simulink model "Main_ekart"  (R2021b)
settings: Solver=FixedStepAuto  StartTime=0.0  StopTime=inf  FixedStep=1/500  RelTol=1e-3  EnableMultiTasking=on
values from neighbouring files (symbols this model uses):
  a = [1 -2.62355180661 2.31468258109 -0.685535977285]    [IMU_filt_100Hz.mat]    (also in IMU_filt_500Hz.mat = [1 -2.92460623545 2.85202781859 -0.92736996835])
  angles = [0 4.9 5 10 15 20 25 30 35 40]    [CreateAllControllers.m]
  b = [0.000699349649901 0.0020980489497 0.0020980489497 0.000699349649901]    [IMU_filt_100Hz.mat]    (also in IMU_filt_500Hz.mat = [6.45184912909e-06 1.93555473873e-05 1.93555473873e-05 6.451)
  D = (DMFx+DMFy)/2    (= 1.2194)    [kart_parameters2.m]
  gear_ratio = 3.2    [kart_parameters2.m]
  L = sys*C    [build_controller_PI.m]    (also in kart_parameters2.m = 1.042)
  newcurrent = [-186.423 -186.283922965 -186.14484593 -186.005768895 -185.866691861 -185.727614826 -185.588537791 -185.449460756 -185.310383721 -185.171306686 -185.032229652 -184.893152617 ... (1000 elements, 1x1000)]    [Torque_map.mat]
  newtorque = [-28.1755 -28.1190925926 -28.0626851852 -28.0062777778 -27.9498703704 -27.893462963 -27.8370555556 -27.7806481481 -27.7242407407 -27.6678333333 -27.6114259259 -27.5550185185 ... (1000 elements, 1x1000)]    [Torque_map.mat]
  percent = [0 0.1001001001 0.2002002002 0.3003003003 0.4004004004 0.500500500501 0.600600600601 0.700700700701 0.800800800801 0.900900900901 1.001001001 1.1011011011 ... (1000 elements, 1x1000)]    [Torque_accel.mat]
  speeds = [0 19.9 20 30 40]    [CreateAllControllers.m]
  table_i = [zeros(1,10) ... (first row only)    [CreateAllControllers.m]
  table_p = [zeros(1, 10) ... (first row only)    [CreateAllControllers.m]
  torque = [0.1025 0.130601101101 0.158702202202 0.186803303303 0.214904404404 0.243005505506 0.271106606607 0.299207707708 0.327308808809 0.35540990991 0.383511011011 0.411612112112 ... (1000 elements, 1x1000)]    [Torque_accel.mat]
libraries: simulink x50, mcp2515lib x46, etargetslib x4, svdutilitieslib x3, cstblocks x2, slpidlib x1
(part 2 of 4)

== system Main_ekart/Receive_CAN/Subsystem6 ==
  CAN_Received : Inport
  CAN_EXT : Inport  Port=2
  CAN_ID : Inport  Port=3
  CAN_DLC : Inport  Port=4
  CAN_DATA : Inport  Port=5
  AND : Logic  Inputs=4  IconShape=distinctive  AllPortsSameDT=off  OutDataTypeStr=boolean
  Compare To Desired DLC : simulink/Logic and Bit Operations/Compare To Constant  relop===  const=DLC  OutDataTypeStr=boolean
  Compare To Desired DLC1 : simulink/Logic and Bit Operations/Compare To Constant  relop===  const=EXT  OutDataTypeStr=boolean
  Compare To Desired ID : simulink/Logic and Bit Operations/Compare To Constant  relop===  const=ID  OutDataTypeStr=boolean
  Memory : Memory
  Switch : Switch  Criteria=u2 > Threshold
  DATA : Outport
  wires:
  CAN_ID/1 -> Compare To Desired ID/1
  CAN_DLC/1 -> Compare To Desired DLC/1
  Compare To Desired DLC/1 -> AND/3
  Compare To Desired ID/1 -> AND/2
  CAN_Received/1 -> AND/1
  AND/1 -> Switch/2
  CAN_DATA/1 -> Switch/1
  Switch/1 -> DATA/1, Memory/1
  Memory/1 -> Switch/3
  CAN_EXT/1 -> Compare To Desired DLC1/1
  Compare To Desired DLC1/1 -> AND/4

== system Main_ekart/Receive_CAN/Subsystem7 ==
  CAN_DATA : Inport
  Byte Unpack : svdutilitieslib/Byte Unpack  dimensions={[1], [1], [1], [1]}  datatypes="{['int16'],  ['int16'], ['int16'], ['int16']}"  byteAlign=1  blockPlatform=arduinoert
      settings: SourceProductBaseCode=ANDROID,ARDUINO,ML_ARDUINO,ECCORTEXA,ECCORTEXR,SC_BEAGLEBONE_BLUE,EC_FREEDOM_BOARD,EC_FRDM_K64F,INTEL_BLOCKSET,MICROBIT,NUCLEO,NVIDIA,PX4AUTOPILOTS,RASPPIIO,STMICRODIS,TIC2000,XILINX_BLOCKSET
  Data Type Conversion : DataTypeConversion  OutDataTypeStr=double
  Data Type Conversion1 : DataTypeConversion  OutDataTypeStr=double
  Data Type Conversion2 : DataTypeConversion  OutDataTypeStr=double
  MATLAB Function : MATLAB Function  TreatAsAtomicUnit=on
  Raw2phys : Gain  Gain=2^(-6)  OutDataTypeStr=Inherit: Inherit via back propagation
  Raw2phys1 : Gain  Gain=2^(-6)  OutDataTypeStr=Inherit: Inherit via back propagation
  Raw2phys2 : Gain  Gain=2^(-6)  OutDataTypeStr=Inherit: Inherit via back propagation
  Terminator : Terminator
  VelX : Outport
  VelY : Outport  Port=2
  VelZ : Outport  Port=3
  wires:
  Raw2phys2/1 -> VelX/1
  Raw2phys1/1 -> VelY/1
  Raw2phys/1 -> VelZ/1
  Byte Unpack/4 -> Data Type Conversion2/1
  Byte Unpack/3 -> Data Type Conversion1/1
  Byte Unpack/2 -> Data Type Conversion/1
  Byte Unpack/1 -> Terminator/1
  MATLAB Function/1(B) -> Byte Unpack/1
  CAN_DATA/1 -> MATLAB Function/1(A)
  Data Type Conversion/1 -> Raw2phys/1
  Data Type Conversion1/1 -> Raw2phys1/1
  Data Type Conversion2/1 -> Raw2phys2/1

== system Main_ekart/CAN send LEFT (Throttle)/CANbegin - WARNING, CONTAINS HARDCODED VALUES/setup ==
  Enable : EnablePort
  CNF1 : Constant  Value=address2A  OutDataTypeStr=uint8
  CNF2 : Constant  Value=address29  OutDataTypeStr=uint8
  CNF3 : Constant  Value=address28  OutDataTypeStr=uint8
  Ground : Ground
  Terminator : Terminator
  changeCANmode(config) : Subsystem  TreatAsAtomicUnit=on
  changeCANmode(normal) : Subsystem  TreatAsAtomicUnit=on
  mcp2515_reset : Subsystem  TreatAsAtomicUnit=on
  setCANRxBuffer : Subsystem  TreatAsAtomicUnit=on
  setCANspeed : Subsystem  TreatAsAtomicUnit=on
  wires:
  CNF3/1 -> setCANspeed/4(CNF3)
  CNF2/1 -> setCANspeed/3(CNF2)
  CNF1/1 -> setCANspeed/2(CNF1)
  mcp2515_reset/1(Out) -> changeCANmode(config)/1(In)
  changeCANmode(config)/1(Out) -> setCANspeed/1(In)
  setCANspeed/1(Out) -> setCANRxBuffer/1(In)
  setCANRxBuffer/1(Out) -> changeCANmode(normal)/1(In)
  Ground/1 -> mcp2515_reset/1(In)
  changeCANmode(normal)/1(Out) -> Terminator/1

== system Main_ekart/CAN send LEFT (Throttle)/CANtransmit/check TxB0 ==
  In1 : Inport
  Bitmask_TxReq : simulink/Logic and Bit Operations/Bitwise Operator  logicop=AND  UseBitMask=on  BitMask=bin2dec('00001000')  BitMaskRealWorld=Stored Integer
  CAN_FAIL : Constant  Value=2  OutDataTypeStr=int8
  CAN_OK : Constant  OutDataTypeStr=int8
  MCP_TxB0CTRL1 : Constant  Value=hex2dec('30')  OutDataTypeStr=uint8
  Switch : Switch  Criteria=u2 > Threshold
  mcp2515_readRegister : Subsystem  TreatAsAtomicUnit=on
  Out1 : Outport  VectorParamsAs1DForOutWhenUnconnected=off
  CANTx_Transmit : Outport  Port=2  VectorParamsAs1DForOutWhenUnconnected=off
  wires:
  CAN_FAIL/1 -> Switch/3
  mcp2515_readRegister/1(Out) -> Out1/1
  mcp2515_readRegister/2(SPI_data) -> Bitmask_TxReq/1
  MCP_TxB0CTRL1/1 -> mcp2515_readRegister/2(address)
  Bitmask_TxReq/1 -> Switch/2
  Switch/1 -> CANTx_Transmit/1
  CAN_OK/1 -> Switch/1
  In1/1 -> mcp2515_readRegister/1(In)

== system Main_ekart/CAN send LEFT (Throttle)/CANtransmit/load Tx data ==
  In1 : Inport
  CAN_ext : Inport  Port=2
  CAN_id : Inport  Port=3
  CAN_dlc : Inport  Port=4
  CAN_data : Inport  Port=5
  MCP_load_TxB0 : Constant  Value=hex2dec('40')  OutDataTypeStr=uint8
  Vector Concatenate : Concatenate  NumInputs=3
  mcp2515_writeTxBuffer : Subsystem  TreatAsAtomicUnit=on
  setID : Subsystem  TreatAsAtomicUnit=on
      settings: RTWSystemCode=Inline
  Out1 : Outport  VectorParamsAs1DForOutWhenUnconnected=off
  wires:
  CAN_ext/1 -> setID/1(ext)
  CAN_id/1 -> setID/2(id)
  CAN_data/1 -> Vector Concatenate/3
  CAN_dlc/1 -> Vector Concatenate/2
  setID/1(TxBn_ID) -> Vector Concatenate/1
  In1/1 -> mcp2515_writeTxBuffer/1(In)
  mcp2515_writeTxBuffer/1(Out) -> Out1/1
  MCP_load_TxB0/1 -> mcp2515_writeTxBuffer/2(cmd_load_tx_buff)
  Vector Concatenate/1 -> mcp2515_writeTxBuffer/3(data_tx_buff)

== system Main_ekart/CAN send LEFT (Throttle)/CANtransmit/send TxB0 ==
  In1 : Inport
  MCP_TxB0CTRL : Constant  Value=hex2dec('30')  OutDataTypeStr=uint8
  TxREQ : Constant  Value=8  OutDataTypeStr=uint8
  mcp2515_writeRegister : Subsystem  TreatAsAtomicUnit=on
  Out1 : Outport  VectorParamsAs1DForOutWhenUnconnected=off
  wires:
  MCP_TxB0CTRL/1 -> mcp2515_writeRegister/2(address)
  mcp2515_writeRegister/1(Out) -> Out1/1
  In1/1 -> mcp2515_writeRegister/1(In)
  TxREQ/1 -> mcp2515_writeRegister/3(value)

== system Main_ekart/CAN send LEFT (brake)/CANbegin - WARNING, CONTAINS HARDCODED VALUES/setup ==
  Enable : EnablePort
  CNF1 : Constant  Value=address2A  OutDataTypeStr=uint8
  CNF2 : Constant  Value=address29  OutDataTypeStr=uint8
  CNF3 : Constant  Value=address28  OutDataTypeStr=uint8
  Ground : Ground
  Terminator : Terminator
  changeCANmode(config) : Subsystem  TreatAsAtomicUnit=on
  changeCANmode(normal) : Subsystem  TreatAsAtomicUnit=on
  mcp2515_reset : Subsystem  TreatAsAtomicUnit=on
  setCANRxBuffer : Subsystem  TreatAsAtomicUnit=on
  setCANspeed : Subsystem  TreatAsAtomicUnit=on
  wires:
  changeCANmode(normal)/1(Out) -> Terminator/1
  Ground/1 -> mcp2515_reset/1(In)
  setCANRxBuffer/1(Out) -> changeCANmode(normal)/1(In)
  setCANspeed/1(Out) -> setCANRxBuffer/1(In)
  changeCANmode(config)/1(Out) -> setCANspeed/1(In)
  mcp2515_reset/1(Out) -> changeCANmode(config)/1(In)
  CNF1/1 -> setCANspeed/2(CNF1)
  CNF2/1 -> setCANspeed/3(CNF2)
  CNF3/1 -> setCANspeed/4(CNF3)

== system Main_ekart/CAN send LEFT (brake)/CANtransmit/check TxB0 ==
  In1 : Inport
  Bitmask_TxReq : simulink/Logic and Bit Operations/Bitwise Operator  logicop=AND  UseBitMask=on  BitMask=bin2dec('00001000')  BitMaskRealWorld=Stored Integer
  CAN_FAIL : Constant  Value=2  OutDataTypeStr=int8
  CAN_OK : Constant  OutDataTypeStr=int8
  MCP_TxB0CTRL1 : Constant  Value=hex2dec('30')  OutDataTypeStr=uint8
  Switch : Switch  Criteria=u2 > Threshold
  mcp2515_readRegister : Subsystem  TreatAsAtomicUnit=on
  Out1 : Outport  VectorParamsAs1DForOutWhenUnconnected=off
  CANTx_Transmit : Outport  Port=2  VectorParamsAs1DForOutWhenUnconnected=off
  wires:
  In1/1 -> mcp2515_readRegister/1(In)
  CAN_OK/1 -> Switch/1
  Switch/1 -> CANTx_Transmit/1
  Bitmask_TxReq/1 -> Switch/2
  MCP_TxB0CTRL1/1 -> mcp2515_readRegister/2(address)
  mcp2515_readRegister/2(SPI_data) -> Bitmask_TxReq/1
  mcp2515_readRegister/1(Out) -> Out1/1
  CAN_FAIL/1 -> Switch/3

== system Main_ekart/CAN send LEFT (brake)/CANtransmit/load Tx data ==
  In1 : Inport
  CAN_ext : Inport  Port=2
  CAN_id : Inport  Port=3
  CAN_dlc : Inport  Port=4
  CAN_data : Inport  Port=5
  MCP_load_TxB0 : Constant  Value=hex2dec('40')  OutDataTypeStr=uint8
  Vector Concatenate : Concatenate  NumInputs=3
  mcp2515_writeTxBuffer : Subsystem  TreatAsAtomicUnit=on
  setID : Subsystem  TreatAsAtomicUnit=on
      settings: RTWSystemCode=Inline
  Out1 : Outport  VectorParamsAs1DForOutWhenUnconnected=off
  wires:
  Vector Concatenate/1 -> mcp2515_writeTxBuffer/3(data_tx_buff)
  MCP_load_TxB0/1 -> mcp2515_writeTxBuffer/2(cmd_load_tx_buff)
  mcp2515_writeTxBuffer/1(Out) -> Out1/1
  In1/1 -> mcp2515_writeTxBuffer/1(In)
  setID/1(TxBn_ID) -> Vector Concatenate/1
  CAN_dlc/1 -> Vector Concatenate/2
  CAN_data/1 -> Vector Concatenate/3
  CAN_id/1 -> setID/2(id)
  CAN_ext/1 -> setID/1(ext)

== system Main_ekart/CAN send LEFT (brake)/CANtransmit/send TxB0 ==
  In1 : Inport
  MCP_TxB0CTRL : Constant  Value=hex2dec('30')  OutDataTypeStr=uint8
  TxREQ : Constant  Value=8  OutDataTypeStr=uint8
  mcp2515_writeRegister : Subsystem  TreatAsAtomicUnit=on
  Out1 : Outport  VectorParamsAs1DForOutWhenUnconnected=off
  wires:
  TxREQ/1 -> mcp2515_writeRegister/3(value)
  In1/1 -> mcp2515_writeRegister/1(In)
  mcp2515_writeRegister/1(Out) -> Out1/1
  MCP_TxB0CTRL/1 -> mcp2515_writeRegister/2(address)

== system Main_ekart/CAN send RIGHT (Brake)/CANbegin - WARNING, CONTAINS HARDCODED VALUES/setup ==
  Enable : EnablePort
  CNF1 : Constant  Value=address2A  OutDataTypeStr=uint8
  CNF2 : Constant  Value=address29  OutDataTypeStr=uint8
  CNF3 : Constant  Value=address28  OutDataTypeStr=uint8
  Ground : Ground
  Terminator : Terminator
  changeCANmode(config) : Subsystem  TreatAsAtomicUnit=on
  changeCANmode(normal) : Subsystem  TreatAsAtomicUnit=on
  mcp2515_reset : Subsystem  TreatAsAtomicUnit=on
  setCANRxBuffer : Subsystem  TreatAsAtomicUnit=on
  setCANspeed : Subsystem  TreatAsAtomicUnit=on
  wires:
  CNF3/1 -> setCANspeed/4(CNF3)
  CNF2/1 -> setCANspeed/3(CNF2)
  CNF1/1 -> setCANspeed/2(CNF1)
  mcp2515_reset/1(Out) -> changeCANmode(config)/1(In)
  changeCANmode(config)/1(Out) -> setCANspeed/1(In)
  setCANspeed/1(Out) -> setCANRxBuffer/1(In)
  setCANRxBuffer/1(Out) -> changeCANmode(normal)/1(In)
  Ground/1 -> mcp2515_reset/1(In)
  changeCANmode(normal)/1(Out) -> Terminator/1

== system Main_ekart/CAN send RIGHT (Brake)/CANtransmit/check TxB0 ==
  In1 : Inport
  Bitmask_TxReq : simulink/Logic and Bit Operations/Bitwise Operator  logicop=AND  UseBitMask=on  BitMask=bin2dec('00001000')  BitMaskRealWorld=Stored Integer
  CAN_FAIL : Constant  Value=2  OutDataTypeStr=int8
  CAN_OK : Constant  OutDataTypeStr=int8
  MCP_TxB0CTRL1 : Constant  Value=hex2dec('30')  OutDataTypeStr=uint8
  Switch : Switch  Criteria=u2 > Threshold
  mcp2515_readRegister : Subsystem  TreatAsAtomicUnit=on
  Out1 : Outport  VectorParamsAs1DForOutWhenUnconnected=off
  CANTx_Transmit : Outport  Port=2  VectorParamsAs1DForOutWhenUnconnected=off
  wires:
  CAN_FAIL/1 -> Switch/3
  mcp2515_readRegister/1(Out) -> Out1/1
  mcp2515_readRegister/2(SPI_data) -> Bitmask_TxReq/1
  MCP_TxB0CTRL1/1 -> mcp2515_readRegister/2(address)
  Bitmask_TxReq/1 -> Switch/2
  Switch/1 -> CANTx_Transmit/1
  CAN_OK/1 -> Switch/1
  In1/1 -> mcp2515_readRegister/1(In)

== system Main_ekart/CAN send RIGHT (Brake)/CANtransmit/load Tx data ==
  In1 : Inport
  CAN_ext : Inport  Port=2
  CAN_id : Inport  Port=3
  CAN_dlc : Inport  Port=4
  CAN_data : Inport  Port=5
  MCP_load_TxB0 : Constant  Value=hex2dec('40')  OutDataTypeStr=uint8
  Vector Concatenate : Concatenate  NumInputs=3
  mcp2515_writeTxBuffer : Subsystem  TreatAsAtomicUnit=on
  setID : Subsystem  TreatAsAtomicUnit=on
      settings: RTWSystemCode=Inline
  Out1 : Outport  VectorParamsAs1DForOutWhenUnconnected=off
  wires:
  CAN_ext/1 -> setID/1(ext)
  CAN_id/1 -> setID/2(id)
  CAN_data/1 -> Vector Concatenate/3
  CAN_dlc/1 -> Vector Concatenate/2
  setID/1(TxBn_ID) -> Vector Concatenate/1
  In1/1 -> mcp2515_writeTxBuffer/1(In)
  mcp2515_writeTxBuffer/1(Out) -> Out1/1
  MCP_load_TxB0/1 -> mcp2515_writeTxBuffer/2(cmd_load_tx_buff)
  Vector Concatenate/1 -> mcp2515_writeTxBuffer/3(data_tx_buff)

== system Main_ekart/CAN send RIGHT (Brake)/CANtransmit/send TxB0 ==
  In1 : Inport
  MCP_TxB0CTRL : Constant  Value=hex2dec('30')  OutDataTypeStr=uint8
  TxREQ : Constant  Value=8  OutDataTypeStr=uint8
  mcp2515_writeRegister : Subsystem  TreatAsAtomicUnit=on
  Out1 : Outport  VectorParamsAs1DForOutWhenUnconnected=off
  wires:
  MCP_TxB0CTRL/1 -> mcp2515_writeRegister/2(address)
  mcp2515_writeRegister/1(Out) -> Out1/1
  In1/1 -> mcp2515_writeRegister/1(In)
  TxREQ/1 -> mcp2515_writeRegister/3(value)

== system Main_ekart/CAN send RIGHT (Throttle)/CANbegin - WARNING, CONTAINS HARDCODED VALUES/setup ==
  Enable : EnablePort
  CNF1 : Constant  Value=address2A  OutDataTypeStr=uint8
  CNF2 : Constant  Value=address29  OutDataTypeStr=uint8
  CNF3 : Constant  Value=address28  OutDataTypeStr=uint8
  Ground : Ground
  Terminator : Terminator
  changeCANmode(config) : Subsystem  TreatAsAtomicUnit=on
  changeCANmode(normal) : Subsystem  TreatAsAtomicUnit=on
  mcp2515_reset : Subsystem  TreatAsAtomicUnit=on
  setCANRxBuffer : Subsystem  TreatAsAtomicUnit=on
  setCANspeed : Subsystem  TreatAsAtomicUnit=on
  wires:
  changeCANmode(normal)/1(Out) -> Terminator/1
  Ground/1 -> mcp2515_reset/1(In)
  setCANRxBuffer/1(Out) -> changeCANmode(normal)/1(In)
  setCANspeed/1(Out) -> setCANRxBuffer/1(In)
  changeCANmode(config)/1(Out) -> setCANspeed/1(In)
  mcp2515_reset/1(Out) -> changeCANmode(config)/1(In)
  CNF1/1 -> setCANspeed/2(CNF1)
  CNF2/1 -> setCANspeed/3(CNF2)
  CNF3/1 -> setCANspeed/4(CNF3)

== system Main_ekart/CAN send RIGHT (Throttle)/CANtransmit/check TxB0 ==
  In1 : Inport
  Bitmask_TxReq : simulink/Logic and Bit Operations/Bitwise Operator  logicop=AND  UseBitMask=on  BitMask=bin2dec('00001000')  BitMaskRealWorld=Stored Integer
  CAN_FAIL : Constant  Value=2  OutDataTypeStr=int8
  CAN_OK : Constant  OutDataTypeStr=int8
  MCP_TxB0CTRL1 : Constant  Value=hex2dec('30')  OutDataTypeStr=uint8
  Switch : Switch  Criteria=u2 > Threshold
  mcp2515_readRegister : Subsystem  TreatAsAtomicUnit=on
  Out1 : Outport  VectorParamsAs1DForOutWhenUnconnected=off
  CANTx_Transmit : Outport  Port=2  VectorParamsAs1DForOutWhenUnconnected=off
  wires:
  In1/1 -> mcp2515_readRegister/1(In)
  CAN_OK/1 -> Switch/1
  Switch/1 -> CANTx_Transmit/1
  Bitmask_TxReq/1 -> Switch/2
  MCP_TxB0CTRL1/1 -> mcp2515_readRegister/2(address)
  mcp2515_readRegister/2(SPI_data) -> Bitmask_TxReq/1
  mcp2515_readRegister/1(Out) -> Out1/1
  CAN_FAIL/1 -> Switch/3

== system Main_ekart/CAN send RIGHT (Throttle)/CANtransmit/load Tx data ==
  In1 : Inport
  CAN_ext : Inport  Port=2
  CAN_id : Inport  Port=3
  CAN_dlc : Inport  Port=4
  CAN_data : Inport  Port=5
  MCP_load_TxB0 : Constant  Value=hex2dec('40')  OutDataTypeStr=uint8
  Vector Concatenate : Concatenate  NumInputs=3
  mcp2515_writeTxBuffer : Subsystem  TreatAsAtomicUnit=on
  setID : Subsystem  TreatAsAtomicUnit=on
      settings: RTWSystemCode=Inline
  Out1 : Outport  VectorParamsAs1DForOutWhenUnconnected=off
  wires:
  Vector Concatenate/1 -> mcp2515_writeTxBuffer/3(data_tx_buff)
  MCP_load_TxB0/1 -> mcp2515_writeTxBuffer/2(cmd_load_tx_buff)
  mcp2515_writeTxBuffer/1(Out) -> Out1/1
  In1/1 -> mcp2515_writeTxBuffer/1(In)
  setID/1(TxBn_ID) -> Vector Concatenate/1
  CAN_dlc/1 -> Vector Concatenate/2
  CAN_data/1 -> Vector Concatenate/3
  CAN_id/1 -> setID/2(id)
  CAN_ext/1 -> setID/1(ext)

== system Main_ekart/CAN send RIGHT (Throttle)/CANtransmit/send TxB0 ==
  In1 : Inport
  MCP_TxB0CTRL : Constant  Value=hex2dec('30')  OutDataTypeStr=uint8
  TxREQ : Constant  Value=8  OutDataTypeStr=uint8
  mcp2515_writeRegister : Subsystem  TreatAsAtomicUnit=on
  Out1 : Outport  VectorParamsAs1DForOutWhenUnconnected=off
  wires:
  TxREQ/1 -> mcp2515_writeRegister/3(value)
  In1/1 -> mcp2515_writeRegister/1(In)
  mcp2515_writeRegister/1(Out) -> Out1/1
  MCP_TxB0CTRL/1 -> mcp2515_writeRegister/2(address)

== system Main_ekart/Receive_CAN/CANreceive/checkRxMsgStatus ==
  RX_STATUS : Inport
  Bitmask_RxBn : simulink/Logic and Bit Operations/Bitwise Operator  logicop=AND  UseBitMask=on  BitMask=bin2dec('11000000')  BitMaskRealWorld=Stored Integer
  CAN_NOMSG : Constant  Value=-1  OutDataTypeStr=int8
  CAN_OK : Constant  OutDataTypeStr=int8
  Switch : Switch  Criteria=u2 > Threshold
  CANRx_Received : Outport
  wires:
  RX_STATUS/1 -> Bitmask_RxBn/1
  CAN_OK/1 -> Switch/1
  CAN_NOMSG/1 -> Switch/3
  Switch/1 -> CANRx_Received/1
  Bitmask_RxBn/1 -> Switch/2

== system Main_ekart/Receive_CAN/CANreceive/mcp2515_read_RX_STATUS ==
  In : Inport
  Constant : Constant  Value=0  OutDataTypeStr=uint8
  MCP_RX_STATUS : Constant  Value=hex2dec('B0')  OutDataTypeStr=uint8
  SPI driver : mcp2515lib/CAN application/mcp2515 driver/SPI driver  SystemSampleTime=-1  VariantActivationTime=update diagram  Latency=0  AutoFrameSizeCalculation=off
      settings: SourceProductName=CAN device driver for mcp2515
  Selector : Selector  IndexMode=Zero-based  InputPortWidth=2  IndexOptions=Index vector (dialog)  Indices=1  OutputSizes=1
  Vector Concatenate : Concatenate
  Out : Outport
  RX_STATUS : Outport  Port=2
  wires:
  In/1 -> Out/1
  Constant/1 -> Vector Concatenate/2
  SPI driver/1 -> Selector/1  "SPIstatus_ext_id"
  Selector/1 -> RX_STATUS/1
  MCP_RX_STATUS/1 -> Vector Concatenate/1
  Vector Concatenate/1 -> SPI driver/1

== system Main_ekart/Receive_CAN/CANreceive/readRxBuffer ==
  RX_STATUS : Inport
  Enable : EnablePort
  Ground : Ground
  Terminator : Terminator
  checkRx1Buffer : Subsystem  TreatAsAtomicUnit=on
  getDLC : Subsystem  TreatAsAtomicUnit=on
  getData : Subsystem  TreatAsAtomicUnit=on
  getID : Subsystem  TreatAsAtomicUnit=on
      settings: RTWSystemCode=Inline
  mcp2515_readRxBuffer : Subsystem  TreatAsAtomicUnit=on
  CAN_ext : Outport
  CAN_id : Outport  Port=2
  CAN_dlc : Outport  Port=3
  CAN_data : Outport  Port=4
  wires:
  getData/1(CAN_data) -> CAN_data/1
  mcp2515_readRxBuffer/2(RxBn) -> getID/1(RxBn), getData/1(RxBx), getDLC/1(RxBx)
  getID/2(CAN_id) -> CAN_id/1
  getID/1(CAN_ext) -> CAN_ext/1
  getDLC/1(CAN_dlc) -> CAN_dlc/1
  mcp2515_readRxBuffer/1(Out) -> Terminator/1
  Ground/1 -> mcp2515_readRxBuffer/1(In)
  RX_STATUS/1 -> checkRx1Buffer/1(RX_STATUS)
  checkRx1Buffer/1(cmd_read_rx_buff) -> mcp2515_readRxBuffer/2(cmd_read_rx_buff)

== system Main_ekart/CAN send LEFT (Throttle)/CANbegin - WARNING, CONTAINS HARDCODED VALUES/setup/changeCANmode(config) ==
  In : Inport
  MCP_CANCTRL : Constant  Value=hex2dec('0F')  OutDataTypeStr=uint8
  MODE_CONFIG : Constant  Value=hex2dec('80')  OutDataTypeStr=uint8
  MODE_MASK : Constant  Value=hex2dec('E0')  OutDataTypeStr=uint8
  mcp2515_modifyRegister : Subsystem  TreatAsAtomicUnit=on
  Out : Outport  VectorParamsAs1DForOutWhenUnconnected=off
  wires:
  MODE_CONFIG/1 -> mcp2515_modifyRegister/4(data)
  MODE_MASK/1 -> mcp2515_modifyRegister/3(mask)
  MCP_CANCTRL/1 -> mcp2515_modifyRegister/2(address)
  In/1 -> mcp2515_modifyRegister/1(In)
  mcp2515_modifyRegister/1(Out) -> Out/1

== system Main_ekart/CAN send LEFT (Throttle)/CANbegin - WARNING, CONTAINS HARDCODED VALUES/setup/changeCANmode(normal) ==
  In : Inport
  MCP_CANCTRL : Constant  Value=hex2dec('0F')  OutDataTypeStr=uint8
  MODE_MASK : Constant  Value=hex2dec('E0')  OutDataTypeStr=uint8
  MODE_NORMAL : Constant  Value=0  OutDataTypeStr=uint8
  mcp2515_modifyRegister : Subsystem  TreatAsAtomicUnit=on
  Out : Outport  VectorParamsAs1DForOutWhenUnconnected=off
  wires:
  MODE_MASK/1 -> mcp2515_modifyRegister/3(mask)
  MODE_NORMAL/1 -> mcp2515_modifyRegister/4(data)
  MCP_CANCTRL/1 -> mcp2515_modifyRegister/2(address)
  In/1 -> mcp2515_modifyRegister/1(In)
  mcp2515_modifyRegister/1(Out) -> Out/1

== system Main_ekart/CAN send LEFT (Throttle)/CANbegin - WARNING, CONTAINS HARDCODED VALUES/setup/mcp2515_reset ==
  In : Inport
  MCP_RESET : Constant  Value=hex2dec('C0')  OutDataTypeStr=uint8
  SPI driver : mcp2515lib/CAN application/mcp2515 driver/SPI driver  SystemSampleTime=-1  VariantActivationTime=update diagram  Latency=0  AutoFrameSizeCalculation=off
      settings: SourceProductName=CAN device driver for mcp2515
  Temporary buffer : DataStoreWrite  DataStoreName=temp_1byte  IndexOptions=Index vector (dialog)  Indices=1  OutputSizes=1
  Out : Outport  VectorParamsAs1DForOutWhenUnconnected=off
  wires:
  MCP_RESET/1 -> SPI driver/1
  In/1 -> Out/1
  SPI driver/1 -> Temporary buffer/1

== system Main_ekart/CAN send LEFT (Throttle)/CANbegin - WARNING, CONTAINS HARDCODED VALUES/setup/setCANRxBuffer ==
  note: RXB0
  note: RXB1
  note: no filter, no mask
  In : Inport
  MCP_RXB0CTRL : Constant  Value=hex2dec('60')  OutDataTypeStr=uint8
  MCP_RXB1CTRL : Constant  Value=hex2dec('70')  OutDataTypeStr=uint8
  MCP_RXB_RX_MASK : Constant  Value=hex2dec('60')  OutDataTypeStr=uint8
  mcp2515_writeRegister : Subsystem  TreatAsAtomicUnit=on
  mcp2515_writeRegister1 : Subsystem  TreatAsAtomicUnit=on
  Out : Outport  VectorParamsAs1DForOutWhenUnconnected=off
  wires:
  MCP_RXB0CTRL/1 -> mcp2515_writeRegister/2(address)
  MCP_RXB1CTRL/1 -> mcp2515_writeRegister1/2(address)
  MCP_RXB_RX_MASK/1 -> mcp2515_writeRegister1/3(value), mcp2515_writeRegister/3(value)
  In/1 -> mcp2515_writeRegister/1(In)
  mcp2515_writeRegister1/1(Out) -> Out/1
  mcp2515_writeRegister/1(Out) -> mcp2515_writeRegister1/1(In)

== system Main_ekart/CAN send LEFT (Throttle)/CANbegin - WARNING, CONTAINS HARDCODED VALUES/setup/setCANspeed ==
  In : Inport
  CNF1 : Inport  Port=2
  CNF2 : Inport  Port=3
  CNF3 : Inport  Port=4
  MCP_CNF1 : Constant  Value=hex2dec('2A')  OutDataTypeStr=uint8
  MCP_CNF2 : Constant  Value=hex2dec('29')  OutDataTypeStr=uint8
  MCP_CNF3 : Constant  Value=hex2dec('28')  OutDataTypeStr=uint8
  mcp2515_writeRegister1 : Subsystem  TreatAsAtomicUnit=on
  mcp2515_writeRegister2 : Subsystem  TreatAsAtomicUnit=on
  mcp2515_writeRegister3 : Subsystem  TreatAsAtomicUnit=on
  Out : Outport  VectorParamsAs1DForOutWhenUnconnected=off
  wires:
  MCP_CNF2/1 -> mcp2515_writeRegister2/2(address)
  MCP_CNF3/1 -> mcp2515_writeRegister3/2(address)
  CNF3/1 -> mcp2515_writeRegister3/3(value)
  CNF1/1 -> mcp2515_writeRegister1/3(value)
  MCP_CNF1/1 -> mcp2515_writeRegister1/2(address)
  CNF2/1 -> mcp2515_writeRegister2/3(value)
  In/1 -> mcp2515_writeRegister1/1(In)
  mcp2515_writeRegister1/1(Out) -> mcp2515_writeRegister2/1(In)
  mcp2515_writeRegister2/1(Out) -> mcp2515_writeRegister3/1(In)
  mcp2515_writeRegister3/1(Out) -> Out/1

== system Main_ekart/CAN send LEFT (Throttle)/CANtransmit/check TxB0/mcp2515_readRegister ==
  In : Inport
  address : Inport  Port=2  OutDataTypeStr=uint8
  Constant : Constant  Value=0  OutDataTypeStr=uint8
  MCP_READ : Constant  Value=3  OutDataTypeStr=uint8
  SPI driver : mcp2515lib/CAN application/mcp2515 driver/SPI driver  SystemSampleTime=-1  VariantActivationTime=update diagram  Latency=0  AutoFrameSizeCalculation=off
      settings: SourceProductName=CAN device driver for mcp2515
  Selector : Selector  IndexMode=Zero-based  InputPortWidth=3  IndexOptions=Index vector (dialog)  Indices=2  OutputSizes=1
  Vector Concatenate : Concatenate  NumInputs=3
  Out : Outport  VectorParamsAs1DForOutWhenUnconnected=off
  SPI_data : Outport  Port=2  VectorParamsAs1DForOutWhenUnconnected=off
  wires:
  SPI driver/1 -> Selector/1
  address/1 -> Vector Concatenate/2
  Constant/1 -> Vector Concatenate/3
  In/1 -> Out/1
  MCP_READ/1 -> Vector Concatenate/1
  Selector/1 -> SPI_data/1
  Vector Concatenate/1 -> SPI driver/1

== system Main_ekart/CAN send LEFT (Throttle)/CANtransmit/load Tx data/mcp2515_writeTxBuffer ==
  In : Inport
  cmd_load_tx_buff : Inport  Port=2
  data_tx_buff : Inport  Port=3
  SPI driver : mcp2515lib/CAN application/mcp2515 driver/SPI driver  SystemSampleTime=-1  VariantActivationTime=update diagram  Latency=0  AutoFrameSizeCalculation=off
      settings: SourceProductName=CAN device driver for mcp2515
  Selector1 : Selector  IndexMode=Zero-based  InputPortWidth=14  IndexOptions=Index vector (dialog)  Indices=0  OutputSizes=1
  Temporary buffer : DataStoreWrite  DataStoreName=temp_1byte  IndexOptions=Index vector (dialog)  Indices=1  OutputSizes=1
  Vector Concatenate : Concatenate
  Out : Outport  VectorParamsAs1DForOutWhenUnconnected=off
  wires:
  In/1 -> Out/1
  SPI driver/1 -> Selector1/1
  data_tx_buff/1 -> Vector Concatenate/2
  cmd_load_tx_buff/1 -> Vector Concatenate/1
  Selector1/1 -> Temporary buffer/1
  Vector Concatenate/1 -> SPI driver/1

== system Main_ekart/CAN send LEFT (Throttle)/CANtransmit/load Tx data/setID ==
  ext : Inport
  id : Inport  Port=2
  Extended ID : Subsystem  TreatAsAtomicUnit=on
  If : If
  Merge : Merge
  Standard ID : Subsystem  TreatAsAtomicUnit=on
  TxBn_ID : Outport  VectorParamsAs1DForOutWhenUnconnected=off
  wires:
  ext/1 -> If/1
  If/1 -> Extended ID/Action
  If/2 -> Standard ID/Action
  Extended ID/1(TxBn_ID) -> Merge/2
  Standard ID/1(TxBn_ID) -> Merge/1
  Merge/1 -> TxBn_ID/1
  id/1 -> Extended ID/1(id), Standard ID/1(id)

== system Main_ekart/CAN send LEFT (Throttle)/CANtransmit/send TxB0/mcp2515_writeRegister ==
  In : Inport
  address : Inport  Port=2  OutDataTypeStr=uint8
  value : Inport  Port=3  OutDataTypeStr=uint8
  MCP_WRITE : Constant  Value=2  OutDataTypeStr=uint8
  SPI driver : mcp2515lib/CAN application/mcp2515 driver/SPI driver  SystemSampleTime=-1  VariantActivationTime=update diagram  Latency=0  AutoFrameSizeCalculation=off
      settings: SourceProductName=CAN device driver for mcp2515
  Selector : Selector  IndexMode=Zero-based  InputPortWidth=3  IndexOptions=Index vector (dialog)  Indices=0  OutputSizes=1
  Temporary buffer : DataStoreWrite  DataStoreName=temp_1byte  IndexOptions=Index vector (dialog)  Indices=1  OutputSizes=1
  Vector Concatenate : Concatenate  NumInputs=3
  Out : Outport  VectorParamsAs1DForOutWhenUnconnected=off
  wires:
  SPI driver/1 -> Selector/1
  Selector/1 -> Temporary buffer/1
  In/1 -> Out/1
  Vector Concatenate/1 -> SPI driver/1
  value/1 -> Vector Concatenate/3
  address/1 -> Vector Concatenate/2
  MCP_WRITE/1 -> Vector Concatenate/1

== system Main_ekart/CAN send LEFT (brake)/CANbegin - WARNING, CONTAINS HARDCODED VALUES/setup/changeCANmode(config) ==
  In : Inport
  MCP_CANCTRL : Constant  Value=hex2dec('0F')  OutDataTypeStr=uint8
  MODE_CONFIG : Constant  Value=hex2dec('80')  OutDataTypeStr=uint8
  MODE_MASK : Constant  Value=hex2dec('E0')  OutDataTypeStr=uint8
  mcp2515_modifyRegister : Subsystem  TreatAsAtomicUnit=on
  Out : Outport  VectorParamsAs1DForOutWhenUnconnected=off
  wires:
  mcp2515_modifyRegister/1(Out) -> Out/1
  In/1 -> mcp2515_modifyRegister/1(In)
  MCP_CANCTRL/1 -> mcp2515_modifyRegister/2(address)
  MODE_MASK/1 -> mcp2515_modifyRegister/3(mask)
  MODE_CONFIG/1 -> mcp2515_modifyRegister/4(data)

== system Main_ekart/CAN send LEFT (brake)/CANbegin - WARNING, CONTAINS HARDCODED VALUES/setup/changeCANmode(normal) ==
  In : Inport
  MCP_CANCTRL : Constant  Value=hex2dec('0F')  OutDataTypeStr=uint8
  MODE_MASK : Constant  Value=hex2dec('E0')  OutDataTypeStr=uint8
  MODE_NORMAL : Constant  Value=0  OutDataTypeStr=uint8
  mcp2515_modifyRegister : Subsystem  TreatAsAtomicUnit=on
  Out : Outport  VectorParamsAs1DForOutWhenUnconnected=off
  wires:
  mcp2515_modifyRegister/1(Out) -> Out/1
  In/1 -> mcp2515_modifyRegister/1(In)
  MCP_CANCTRL/1 -> mcp2515_modifyRegister/2(address)
  MODE_NORMAL/1 -> mcp2515_modifyRegister/4(data)
  MODE_MASK/1 -> mcp2515_modifyRegister/3(mask)

== system Main_ekart/CAN send LEFT (brake)/CANbegin - WARNING, CONTAINS HARDCODED VALUES/setup/mcp2515_reset ==
  In : Inport
  MCP_RESET : Constant  Value=hex2dec('C0')  OutDataTypeStr=uint8
  SPI driver : mcp2515lib/CAN application/mcp2515 driver/SPI driver  SystemSampleTime=-1  VariantActivationTime=update diagram  Latency=0  AutoFrameSizeCalculation=off
      settings: SourceProductName=CAN device driver for mcp2515
  Temporary buffer : DataStoreWrite  DataStoreName=temp_1byte  IndexOptions=Index vector (dialog)  Indices=1  OutputSizes=1
  Out : Outport  VectorParamsAs1DForOutWhenUnconnected=off
  wires:
  SPI driver/1 -> Temporary buffer/1
  In/1 -> Out/1
  MCP_RESET/1 -> SPI driver/1

== system Main_ekart/CAN send LEFT (brake)/CANbegin - WARNING, CONTAINS HARDCODED VALUES/setup/setCANRxBuffer ==
  note: no filter, no mask
  note: RXB1
  note: RXB0
  In : Inport
  MCP_RXB0CTRL : Constant  Value=hex2dec('60')  OutDataTypeStr=uint8
  MCP_RXB1CTRL : Constant  Value=hex2dec('70')  OutDataTypeStr=uint8
  MCP_RXB_RX_MASK : Constant  Value=hex2dec('60')  OutDataTypeStr=uint8
  mcp2515_writeRegister : Subsystem  TreatAsAtomicUnit=on
  mcp2515_writeRegister1 : Subsystem  TreatAsAtomicUnit=on
  Out : Outport  VectorParamsAs1DForOutWhenUnconnected=off
  wires:
  mcp2515_writeRegister/1(Out) -> mcp2515_writeRegister1/1(In)
  mcp2515_writeRegister1/1(Out) -> Out/1
  In/1 -> mcp2515_writeRegister/1(In)
  MCP_RXB_RX_MASK/1 -> mcp2515_writeRegister/3(value), mcp2515_writeRegister1/3(value)
  MCP_RXB1CTRL/1 -> mcp2515_writeRegister1/2(address)
  MCP_RXB0CTRL/1 -> mcp2515_writeRegister/2(address)

== system Main_ekart/CAN send LEFT (brake)/CANbegin - WARNING, CONTAINS HARDCODED VALUES/setup/setCANspeed ==
  In : Inport
  CNF1 : Inport  Port=2
  CNF2 : Inport  Port=3
  CNF3 : Inport  Port=4
  MCP_CNF1 : Constant  Value=hex2dec('2A')  OutDataTypeStr=uint8
  MCP_CNF2 : Constant  Value=hex2dec('29')  OutDataTypeStr=uint8
  MCP_CNF3 : Constant  Value=hex2dec('28')  OutDataTypeStr=uint8
  mcp2515_writeRegister1 : Subsystem  TreatAsAtomicUnit=on
  mcp2515_writeRegister2 : Subsystem  TreatAsAtomicUnit=on
  mcp2515_writeRegister3 : Subsystem  TreatAsAtomicUnit=on
  Out : Outport  VectorParamsAs1DForOutWhenUnconnected=off
  wires:
  mcp2515_writeRegister3/1(Out) -> Out/1
  mcp2515_writeRegister2/1(Out) -> mcp2515_writeRegister3/1(In)
  mcp2515_writeRegister1/1(Out) -> mcp2515_writeRegister2/1(In)
  In/1 -> mcp2515_writeRegister1/1(In)
  CNF2/1 -> mcp2515_writeRegister2/3(value)
  MCP_CNF1/1 -> mcp2515_writeRegister1/2(address)
  CNF1/1 -> mcp2515_writeRegister1/3(value)
  CNF3/1 -> mcp2515_writeRegister3/3(value)
  MCP_CNF3/1 -> mcp2515_writeRegister3/2(address)
  MCP_CNF2/1 -> mcp2515_writeRegister2/2(address)

== system Main_ekart/CAN send LEFT (brake)/CANtransmit/check TxB0/mcp2515_readRegister ==
  In : Inport
  address : Inport  Port=2  OutDataTypeStr=uint8
  Constant : Constant  Value=0  OutDataTypeStr=uint8
  MCP_READ : Constant  Value=3  OutDataTypeStr=uint8
  SPI driver : mcp2515lib/CAN application/mcp2515 driver/SPI driver  SystemSampleTime=-1  VariantActivationTime=update diagram  Latency=0  AutoFrameSizeCalculation=off
      settings: SourceProductName=CAN device driver for mcp2515
  Selector : Selector  IndexMode=Zero-based  InputPortWidth=3  IndexOptions=Index vector (dialog)  Indices=2  OutputSizes=1
  Vector Concatenate : Concatenate  NumInputs=3
  Out : Outport  VectorParamsAs1DForOutWhenUnconnected=off
  SPI_data : Outport  Port=2  VectorParamsAs1DForOutWhenUnconnected=off
  wires:
  Vector Concatenate/1 -> SPI driver/1
  Selector/1 -> SPI_data/1
  MCP_READ/1 -> Vector Concatenate/1
  In/1 -> Out/1
  Constant/1 -> Vector Concatenate/3
  address/1 -> Vector Concatenate/2
  SPI driver/1 -> Selector/1

== system Main_ekart/CAN send LEFT (brake)/CANtransmit/load Tx data/mcp2515_writeTxBuffer ==
  In : Inport
  cmd_load_tx_buff : Inport  Port=2
  data_tx_buff : Inport  Port=3
  SPI driver : mcp2515lib/CAN application/mcp2515 driver/SPI driver  SystemSampleTime=-1  VariantActivationTime=update diagram  Latency=0  AutoFrameSizeCalculation=off
      settings: SourceProductName=CAN device driver for mcp2515
  Selector1 : Selector  IndexMode=Zero-based  InputPortWidth=14  IndexOptions=Index vector (dialog)  Indices=0  OutputSizes=1
  Temporary buffer : DataStoreWrite  DataStoreName=temp_1byte  IndexOptions=Index vector (dialog)  Indices=1  OutputSizes=1
  Vector Concatenate : Concatenate
  Out : Outport  VectorParamsAs1DForOutWhenUnconnected=off
  wires:
  Vector Concatenate/1 -> SPI driver/1
  Selector1/1 -> Temporary buffer/1
  cmd_load_tx_buff/1 -> Vector Concatenate/1
  data_tx_buff/1 -> Vector Concatenate/2
  SPI driver/1 -> Selector1/1
  In/1 -> Out/1

== system Main_ekart/CAN send LEFT (brake)/CANtransmit/load Tx data/setID ==
  ext : Inport
  id : Inport  Port=2
  Extended ID : Subsystem  TreatAsAtomicUnit=on
  If : If
  Merge : Merge
  Standard ID : Subsystem  TreatAsAtomicUnit=on
  TxBn_ID : Outport  VectorParamsAs1DForOutWhenUnconnected=off
  wires:
  id/1 -> Standard ID/1(id), Extended ID/1(id)
  Merge/1 -> TxBn_ID/1
  Standard ID/1(TxBn_ID) -> Merge/1
  Extended ID/1(TxBn_ID) -> Merge/2
  If/2 -> Standard ID/Action
  If/1 -> Extended ID/Action
  ext/1 -> If/1

== system Main_ekart/CAN send LEFT (brake)/CANtransmit/send TxB0/mcp2515_writeRegister ==
  In : Inport
  address : Inport  Port=2  OutDataTypeStr=uint8
  value : Inport  Port=3  OutDataTypeStr=uint8
  MCP_WRITE : Constant  Value=2  OutDataTypeStr=uint8
  SPI driver : mcp2515lib/CAN application/mcp2515 driver/SPI driver  SystemSampleTime=-1  VariantActivationTime=update diagram  Latency=0  AutoFrameSizeCalculation=off
      settings: SourceProductName=CAN device driver for mcp2515
  Selector : Selector  IndexMode=Zero-based  InputPortWidth=3  IndexOptions=Index vector (dialog)  Indices=0  OutputSizes=1
  Temporary buffer : DataStoreWrite  DataStoreName=temp_1byte  IndexOptions=Index vector (dialog)  Indices=1  OutputSizes=1
  Vector Concatenate : Concatenate  NumInputs=3
  Out : Outport  VectorParamsAs1DForOutWhenUnconnected=off
  wires:
  MCP_WRITE/1 -> Vector Concatenate/1
  address/1 -> Vector Concatenate/2
  value/1 -> Vector Concatenate/3
  Vector Concatenate/1 -> SPI driver/1
  In/1 -> Out/1
  Selector/1 -> Temporary buffer/1
  SPI driver/1 -> Selector/1

== system Main_ekart/CAN send RIGHT (Brake)/CANbegin - WARNING, CONTAINS HARDCODED VALUES/setup/changeCANmode(config) ==
  In : Inport
  MCP_CANCTRL : Constant  Value=hex2dec('0F')  OutDataTypeStr=uint8
  MODE_CONFIG : Constant  Value=hex2dec('80')  OutDataTypeStr=uint8
  MODE_MASK : Constant  Value=hex2dec('E0')  OutDataTypeStr=uint8
  mcp2515_modifyRegister : Subsystem  TreatAsAtomicUnit=on
  Out : Outport  VectorParamsAs1DForOutWhenUnconnected=off
  wires:
  MODE_CONFIG/1 -> mcp2515_modifyRegister/4(data)
  MODE_MASK/1 -> mcp2515_modifyRegister/3(mask)
  MCP_CANCTRL/1 -> mcp2515_modifyRegister/2(address)
  In/1 -> mcp2515_modifyRegister/1(In)
  mcp2515_modifyRegister/1(Out) -> Out/1

== system Main_ekart/CAN send RIGHT (Brake)/CANbegin - WARNING, CONTAINS HARDCODED VALUES/setup/changeCANmode(normal) ==
  In : Inport
  MCP_CANCTRL : Constant  Value=hex2dec('0F')  OutDataTypeStr=uint8
  MODE_MASK : Constant  Value=hex2dec('E0')  OutDataTypeStr=uint8
  MODE_NORMAL : Constant  Value=0  OutDataTypeStr=uint8
  mcp2515_modifyRegister : Subsystem  TreatAsAtomicUnit=on
  Out : Outport  VectorParamsAs1DForOutWhenUnconnected=off
  wires:
  MODE_MASK/1 -> mcp2515_modifyRegister/3(mask)
  MODE_NORMAL/1 -> mcp2515_modifyRegister/4(data)
  MCP_CANCTRL/1 -> mcp2515_modifyRegister/2(address)
  In/1 -> mcp2515_modifyRegister/1(In)
  mcp2515_modifyRegister/1(Out) -> Out/1

== system Main_ekart/CAN send RIGHT (Brake)/CANbegin - WARNING, CONTAINS HARDCODED VALUES/setup/mcp2515_reset ==
  In : Inport
  MCP_RESET : Constant  Value=hex2dec('C0')  OutDataTypeStr=uint8
  SPI driver : mcp2515lib/CAN application/mcp2515 driver/SPI driver  SystemSampleTime=-1  VariantActivationTime=update diagram  Latency=0  AutoFrameSizeCalculation=off
      settings: SourceProductName=CAN device driver for mcp2515
  Temporary buffer : DataStoreWrite  DataStoreName=temp_1byte  IndexOptions=Index vector (dialog)  Indices=1  OutputSizes=1
  Out : Outport  VectorParamsAs1DForOutWhenUnconnected=off
  wires:
  MCP_RESET/1 -> SPI driver/1
  In/1 -> Out/1
  SPI driver/1 -> Temporary buffer/1

== system Main_ekart/CAN send RIGHT (Brake)/CANbegin - WARNING, CONTAINS HARDCODED VALUES/setup/setCANRxBuffer ==
  note: RXB0
  note: RXB1
  note: no filter, no mask
  In : Inport
  MCP_RXB0CTRL : Constant  Value=hex2dec('60')  OutDataTypeStr=uint8
  MCP_RXB1CTRL : Constant  Value=hex2dec('70')  OutDataTypeStr=uint8
  MCP_RXB_RX_MASK : Constant  Value=hex2dec('60')  OutDataTypeStr=uint8
  mcp2515_writeRegister : Subsystem  TreatAsAtomicUnit=on
  mcp2515_writeRegister1 : Subsystem  TreatAsAtomicUnit=on
  Out : Outport  VectorParamsAs1DForOutWhenUnconnected=off
  wires:
  MCP_RXB0CTRL/1 -> mcp2515_writeRegister/2(address)
  MCP_RXB1CTRL/1 -> mcp2515_writeRegister1/2(address)
  MCP_RXB_RX_MASK/1 -> mcp2515_writeRegister1/3(value), mcp2515_writeRegister/3(value)
  In/1 -> mcp2515_writeRegister/1(In)
  mcp2515_writeRegister1/1(Out) -> Out/1
  mcp2515_writeRegister/1(Out) -> mcp2515_writeRegister1/1(In)

== system Main_ekart/CAN send RIGHT (Brake)/CANbegin - WARNING, CONTAINS HARDCODED VALUES/setup/setCANspeed ==
  In : Inport
  CNF1 : Inport  Port=2
  CNF2 : Inport  Port=3
  CNF3 : Inport  Port=4
  MCP_CNF1 : Constant  Value=hex2dec('2A')  OutDataTypeStr=uint8
  MCP_CNF2 : Constant  Value=hex2dec('29')  OutDataTypeStr=uint8
  MCP_CNF3 : Constant  Value=hex2dec('28')  OutDataTypeStr=uint8
  mcp2515_writeRegister1 : Subsystem  TreatAsAtomicUnit=on
  mcp2515_writeRegister2 : Subsystem  TreatAsAtomicUnit=on
  mcp2515_writeRegister3 : Subsystem  TreatAsAtomicUnit=on
  Out : Outport  VectorParamsAs1DForOutWhenUnconnected=off
  wires:
  MCP_CNF2/1 -> mcp2515_writeRegister2/2(address)
  MCP_CNF3/1 -> mcp2515_writeRegister3/2(address)
  CNF3/1 -> mcp2515_writeRegister3/3(value)
  CNF1/1 -> mcp2515_writeRegister1/3(value)
  MCP_CNF1/1 -> mcp2515_writeRegister1/2(address)
  CNF2/1 -> mcp2515_writeRegister2/3(value)
  In/1 -> mcp2515_writeRegister1/1(In)
  mcp2515_writeRegister1/1(Out) -> mcp2515_writeRegister2/1(In)
  mcp2515_writeRegister2/1(Out) -> mcp2515_writeRegister3/1(In)
  mcp2515_writeRegister3/1(Out) -> Out/1

== system Main_ekart/CAN send RIGHT (Brake)/CANtransmit/check TxB0/mcp2515_readRegister ==
  In : Inport
  address : Inport  Port=2  OutDataTypeStr=uint8
  Constant : Constant  Value=0  OutDataTypeStr=uint8
  MCP_READ : Constant  Value=3  OutDataTypeStr=uint8
  SPI driver : mcp2515lib/CAN application/mcp2515 driver/SPI driver  SystemSampleTime=-1  VariantActivationTime=update diagram  Latency=0  AutoFrameSizeCalculation=off
      settings: SourceProductName=CAN device driver for mcp2515
  Selector : Selector  IndexMode=Zero-based  InputPortWidth=3  IndexOptions=Index vector (dialog)  Indices=2  OutputSizes=1
  Vector Concatenate : Concatenate  NumInputs=3
  Out : Outport  VectorParamsAs1DForOutWhenUnconnected=off
  SPI_data : Outport  Port=2  VectorParamsAs1DForOutWhenUnconnected=off
  wires:
  SPI driver/1 -> Selector/1
  address/1 -> Vector Concatenate/2
  Constant/1 -> Vector Concatenate/3
  In/1 -> Out/1
  MCP_READ/1 -> Vector Concatenate/1
  Selector/1 -> SPI_data/1
  Vector Concatenate/1 -> SPI driver/1

== system Main_ekart/CAN send RIGHT (Brake)/CANtransmit/load Tx data/mcp2515_writeTxBuffer ==
  In : Inport
  cmd_load_tx_buff : Inport  Port=2
  data_tx_buff : Inport  Port=3
  SPI driver : mcp2515lib/CAN application/mcp2515 driver/SPI driver  SystemSampleTime=-1  VariantActivationTime=update diagram  Latency=0  AutoFrameSizeCalculation=off
      settings: SourceProductName=CAN device driver for mcp2515
  Selector1 : Selector  IndexMode=Zero-based  InputPortWidth=14  IndexOptions=Index vector (dialog)  Indices=0  OutputSizes=1
  Temporary buffer : DataStoreWrite  DataStoreName=temp_1byte  IndexOptions=Index vector (dialog)  Indices=1  OutputSizes=1
  Vector Concatenate : Concatenate
  Out : Outport  VectorParamsAs1DForOutWhenUnconnected=off
  wires:
  In/1 -> Out/1
  SPI driver/1 -> Selector1/1
  data_tx_buff/1 -> Vector Concatenate/2
  cmd_load_tx_buff/1 -> Vector Concatenate/1
  Selector1/1 -> Temporary buffer/1
  Vector Concatenate/1 -> SPI driver/1

== system Main_ekart/CAN send RIGHT (Brake)/CANtransmit/load Tx data/setID ==
  ext : Inport
  id : Inport  Port=2
  Extended ID : Subsystem  TreatAsAtomicUnit=on
  If : If
  Merge : Merge
  Standard ID : Subsystem  TreatAsAtomicUnit=on
  TxBn_ID : Outport  VectorParamsAs1DForOutWhenUnconnected=off
  wires:
  ext/1 -> If/1
  If/1 -> Extended ID/Action
  If/2 -> Standard ID/Action
  Extended ID/1(TxBn_ID) -> Merge/2
  Standard ID/1(TxBn_ID) -> Merge/1
  Merge/1 -> TxBn_ID/1
  id/1 -> Extended ID/1(id), Standard ID/1(id)

== system Main_ekart/CAN send RIGHT (Brake)/CANtransmit/send TxB0/mcp2515_writeRegister ==
  In : Inport
  address : Inport  Port=2  OutDataTypeStr=uint8
  value : Inport  Port=3  OutDataTypeStr=uint8
  MCP_WRITE : Constant  Value=2  OutDataTypeStr=uint8
  SPI driver : mcp2515lib/CAN application/mcp2515 driver/SPI driver  SystemSampleTime=-1  VariantActivationTime=update diagram  Latency=0  AutoFrameSizeCalculation=off
      settings: SourceProductName=CAN device driver for mcp2515
  Selector : Selector  IndexMode=Zero-based  InputPortWidth=3  IndexOptions=Index vector (dialog)  Indices=0  OutputSizes=1
  Temporary buffer : DataStoreWrite  DataStoreName=temp_1byte  IndexOptions=Index vector (dialog)  Indices=1  OutputSizes=1
  Vector Concatenate : Concatenate  NumInputs=3
  Out : Outport  VectorParamsAs1DForOutWhenUnconnected=off
  wires:
  SPI driver/1 -> Selector/1
  Selector/1 -> Temporary buffer/1
  In/1 -> Out/1
  Vector Concatenate/1 -> SPI driver/1
  value/1 -> Vector Concatenate/3
  address/1 -> Vector Concatenate/2
  MCP_WRITE/1 -> Vector Concatenate/1

== system Main_ekart/CAN send RIGHT (Throttle)/CANbegin - WARNING, CONTAINS HARDCODED VALUES/setup/changeCANmode(config) ==
  In : Inport
  MCP_CANCTRL : Constant  Value=hex2dec('0F')  OutDataTypeStr=uint8
  MODE_CONFIG : Constant  Value=hex2dec('80')  OutDataTypeStr=uint8
  MODE_MASK : Constant  Value=hex2dec('E0')  OutDataTypeStr=uint8
  mcp2515_modifyRegister : Subsystem  TreatAsAtomicUnit=on
  Out : Outport  VectorParamsAs1DForOutWhenUnconnected=off
  wires:
  mcp2515_modifyRegister/1(Out) -> Out/1
  In/1 -> mcp2515_modifyRegister/1(In)
  MCP_CANCTRL/1 -> mcp2515_modifyRegister/2(address)
  MODE_MASK/1 -> mcp2515_modifyRegister/3(mask)
  MODE_CONFIG/1 -> mcp2515_modifyRegister/4(data)

== system Main_ekart/CAN send RIGHT (Throttle)/CANbegin - WARNING, CONTAINS HARDCODED VALUES/setup/changeCANmode(normal) ==
  In : Inport
  MCP_CANCTRL : Constant  Value=hex2dec('0F')  OutDataTypeStr=uint8
  MODE_MASK : Constant  Value=hex2dec('E0')  OutDataTypeStr=uint8
  MODE_NORMAL : Constant  Value=0  OutDataTypeStr=uint8
  mcp2515_modifyRegister : Subsystem  TreatAsAtomicUnit=on
  Out : Outport  VectorParamsAs1DForOutWhenUnconnected=off
  wires:
  mcp2515_modifyRegister/1(Out) -> Out/1
  In/1 -> mcp2515_modifyRegister/1(In)
  MCP_CANCTRL/1 -> mcp2515_modifyRegister/2(address)
  MODE_NORMAL/1 -> mcp2515_modifyRegister/4(data)
  MODE_MASK/1 -> mcp2515_modifyRegister/3(mask)

== system Main_ekart/CAN send RIGHT (Throttle)/CANbegin - WARNING, CONTAINS HARDCODED VALUES/setup/mcp2515_reset ==
  In : Inport
  MCP_RESET : Constant  Value=hex2dec('C0')  OutDataTypeStr=uint8
  SPI driver : mcp2515lib/CAN application/mcp2515 driver/SPI driver  SystemSampleTime=-1  VariantActivationTime=update diagram  Latency=0  AutoFrameSizeCalculation=off
      settings: SourceProductName=CAN device driver for mcp2515
  Temporary buffer : DataStoreWrite  DataStoreName=temp_1byte  IndexOptions=Index vector (dialog)  Indices=1  OutputSizes=1
  Out : Outport  VectorParamsAs1DForOutWhenUnconnected=off
  wires:
  SPI driver/1 -> Temporary buffer/1
  In/1 -> Out/1
  MCP_RESET/1 -> SPI driver/1

== system Main_ekart/CAN send RIGHT (Throttle)/CANbegin - WARNING, CONTAINS HARDCODED VALUES/setup/setCANRxBuffer ==
  note: no filter, no mask
  note: RXB1
  note: RXB0
  In : Inport
  MCP_RXB0CTRL : Constant  Value=hex2dec('60')  OutDataTypeStr=uint8
  MCP_RXB1CTRL : Constant  Value=hex2dec('70')  OutDataTypeStr=uint8
  MCP_RXB_RX_MASK : Constant  Value=hex2dec('60')  OutDataTypeStr=uint8
  mcp2515_writeRegister : Subsystem  TreatAsAtomicUnit=on
  mcp2515_writeRegister1 : Subsystem  TreatAsAtomicUnit=on
  Out : Outport  VectorParamsAs1DForOutWhenUnconnected=off
  wires:
  mcp2515_writeRegister/1(Out) -> mcp2515_writeRegister1/1(In)
  mcp2515_writeRegister1/1(Out) -> Out/1
  In/1 -> mcp2515_writeRegister/1(In)
  MCP_RXB_RX_MASK/1 -> mcp2515_writeRegister/3(value), mcp2515_writeRegister1/3(value)
  MCP_RXB1CTRL/1 -> mcp2515_writeRegister1/2(address)
  MCP_RXB0CTRL/1 -> mcp2515_writeRegister/2(address)

== system Main_ekart/CAN send RIGHT (Throttle)/CANbegin - WARNING, CONTAINS HARDCODED VALUES/setup/setCANspeed ==
  In : Inport
  CNF1 : Inport  Port=2
  CNF2 : Inport  Port=3
  CNF3 : Inport  Port=4
  MCP_CNF1 : Constant  Value=hex2dec('2A')  OutDataTypeStr=uint8
  MCP_CNF2 : Constant  Value=hex2dec('29')  OutDataTypeStr=uint8
  MCP_CNF3 : Constant  Value=hex2dec('28')  OutDataTypeStr=uint8
  mcp2515_writeRegister1 : Subsystem  TreatAsAtomicUnit=on
  mcp2515_writeRegister2 : Subsystem  TreatAsAtomicUnit=on
  mcp2515_writeRegister3 : Subsystem  TreatAsAtomicUnit=on
  Out : Outport  VectorParamsAs1DForOutWhenUnconnected=off
  wires:
  mcp2515_writeRegister3/1(Out) -> Out/1
  mcp2515_writeRegister2/1(Out) -> mcp2515_writeRegister3/1(In)
  mcp2515_writeRegister1/1(Out) -> mcp2515_writeRegister2/1(In)
  In/1 -> mcp2515_writeRegister1/1(In)
  CNF2/1 -> mcp2515_writeRegister2/3(value)
  MCP_CNF1/1 -> mcp2515_writeRegister1/2(address)
  CNF1/1 -> mcp2515_writeRegister1/3(value)
  CNF3/1 -> mcp2515_writeRegister3/3(value)
  MCP_CNF3/1 -> mcp2515_writeRegister3/2(address)
  MCP_CNF2/1 -> mcp2515_writeRegister2/2(address)

== system Main_ekart/CAN send RIGHT (Throttle)/CANtransmit/check TxB0/mcp2515_readRegister ==
  In : Inport
  address : Inport  Port=2  OutDataTypeStr=uint8
  Constant : Constant  Value=0  OutDataTypeStr=uint8
  MCP_READ : Constant  Value=3  OutDataTypeStr=uint8
  SPI driver : mcp2515lib/CAN application/mcp2515 driver/SPI driver  SystemSampleTime=-1  VariantActivationTime=update diagram  Latency=0  AutoFrameSizeCalculation=off
      settings: SourceProductName=CAN device driver for mcp2515
  Selector : Selector  IndexMode=Zero-based  InputPortWidth=3  IndexOptions=Index vector (dialog)  Indices=2  OutputSizes=1
  Vector Concatenate : Concatenate  NumInputs=3
  Out : Outport  VectorParamsAs1DForOutWhenUnconnected=off
  SPI_data : Outport  Port=2  VectorParamsAs1DForOutWhenUnconnected=off
  wires:
  Vector Concatenate/1 -> SPI driver/1
  Selector/1 -> SPI_data/1
  MCP_READ/1 -> Vector Concatenate/1
  In/1 -> Out/1
  Constant/1 -> Vector Concatenate/3
  address/1 -> Vector Concatenate/2
  SPI driver/1 -> Selector/1

== system Main_ekart/CAN send RIGHT (Throttle)/CANtransmit/load Tx data/mcp2515_writeTxBuffer ==
  In : Inport
  cmd_load_tx_buff : Inport  Port=2
  data_tx_buff : Inport  Port=3
  SPI driver : mcp2515lib/CAN application/mcp2515 driver/SPI driver  SystemSampleTime=-1  VariantActivationTime=update diagram  Latency=0  AutoFrameSizeCalculation=off
      settings: SourceProductName=CAN device driver for mcp2515
  Selector1 : Selector  IndexMode=Zero-based  InputPortWidth=14  IndexOptions=Index vector (dialog)  Indices=0  OutputSizes=1
  Temporary buffer : DataStoreWrite  DataStoreName=temp_1byte  IndexOptions=Index vector (dialog)  Indices=1  OutputSizes=1
  Vector Concatenate : Concatenate
  Out : Outport  VectorParamsAs1DForOutWhenUnconnected=off
  wires:
  Vector Concatenate/1 -> SPI driver/1
  Selector1/1 -> Temporary buffer/1
  cmd_load_tx_buff/1 -> Vector Concatenate/1
  data_tx_buff/1 -> Vector Concatenate/2
  SPI driver/1 -> Selector1/1
  In/1 -> Out/1
